simulink model "FOSWEC_flapForcedOscillation"  (R2014b)
settings: Solver=ode4  StartTime=0  StopTime=100  FixedStep=0.05  RelTol=1e-3
undefined symbols (not defined in the file or in its folder): body, constraint, pto
libraries: WECSim_Lib x15
settings Model: Creator=cmichel  LastModifiedBy=cmichel

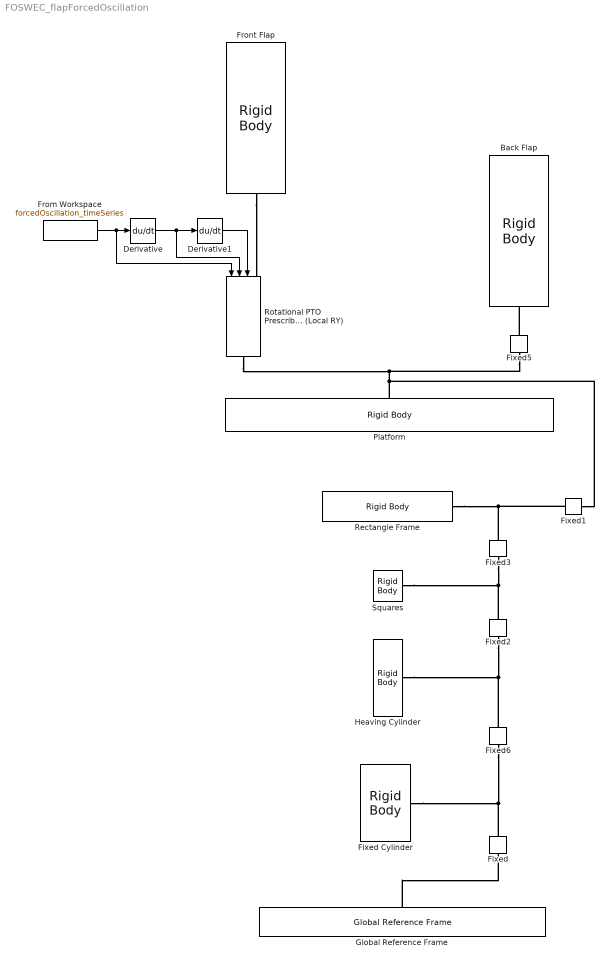
== system FOSWEC_flapForcedOscillation ==
  Back Flap : WECSim_Lib/Body Elements/Rigid Body  body=body(3)
      settings: AttributesFormatString=%<body>
  Derivative : Derivative
  Derivative1 : Derivative
  Fixed : WECSim_Lib/Constraints/Fixed  constraint=constraint(5)
      settings: AttributesFormatString=%<constraint>
  Fixed Cylinder : WECSim_Lib/Body Elements/Rigid Body  body=body(7)
      settings: AttributesFormatString=%<body>
  Fixed1 : WECSim_Lib/Constraints/Fixed  constraint=constraint(1)
      settings: AttributesFormatString=%<constraint>
  Fixed2 : WECSim_Lib/Constraints/Fixed  constraint=constraint(3)
      settings: AttributesFormatString=%<constraint>
  Fixed3 : WECSim_Lib/Constraints/Fixed  constraint=constraint(2)
      settings: AttributesFormatString=%<constraint>
  Fixed5 : WECSim_Lib/Constraints/Fixed  constraint=constraint(6)
      settings: AttributesFormatString=%<constraint>
  Fixed6 : WECSim_Lib/Constraints/Fixed  constraint=constraint(4)
      settings: AttributesFormatString=%<constraint>
  From Workspace : FromWorkspace  VariableName=forcedOscillation_timeSeries  SampleTime=0
  Front Flap : WECSim_Lib/Body Elements/Rigid Body  body=body(2)
      settings: AttributesFormatString=%<body>
  Global Reference Frame : WECSim_Lib/Frames/Global Reference Frame  waves=waves  simu=simu
  Heaving Cylinder : WECSim_Lib/Body Elements/Rigid Body  body=body(6)
      settings: AttributesFormatString=%<body>
  Platform : WECSim_Lib/Body Elements/Rigid Body  body=body(1)
      settings: AttributesFormatString=%<body>
  Rectangle Frame : WECSim_Lib/Body Elements/Rigid Body  body=body(4)
      settings: AttributesFormatString=%<body>
  Rotational PTO Prescribed Motion (Local RY) : WECSim_Lib/PTOs/Rotational PTO Prescribed Motion (Local RY)  pto=pto(1)
      settings: AttributesFormatString=%<pto>
  Squares : WECSim_Lib/Body Elements/Rigid Body  body=body(5)
      settings: AttributesFormatString=%<body>
  wires:
  From Workspace/1 -> Derivative/1, Rotational PTO Prescribed Motion (Local RY)/1
  Derivative/1 -> Rotational PTO Prescribed Motion (Local RY)/2, Derivative1/1
  Derivative1/1 -> Rotational PTO Prescribed Motion (Local RY)/3
  connections:
  Fixed5/RConn1 -- Back Flap/RConn1
  Platform/RConn1 -- Rotational PTO Prescribed Motion (Local RY)/RConn1 -- Fixed5/LConn1 -- Fixed1/RConn1
  Global Reference Frame/RConn1 -- Fixed/LConn1
  Fixed3/LConn1 -- Fixed2/RConn1 -- Squares/RConn1
  Fixed1/LConn1 -- Fixed3/RConn1 -- Rectangle Frame/RConn1
  Fixed6/RConn1 -- Fixed2/LConn1 -- Heaving Cylinder/RConn1
  Fixed6/LConn1 -- Fixed Cylinder/RConn1 -- Fixed/RConn1
  Front Flap/RConn1 -- Rotational PTO Prescribed Motion (Local RY)/LConn1
